simulink model "task_5_model"  (R2021b)
settings: Solver=FixedStepAuto  StartTime=0.0  StopTime=2  FixedStep=0.001  RelTol=1e-3
settings Model: Creator=den  LastModifiedBy=den

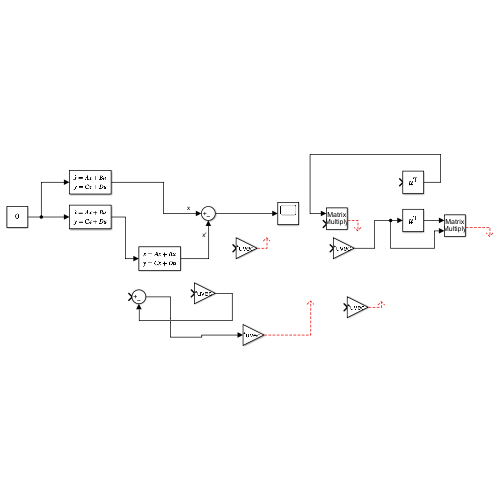
[thumbnail: Simulink's stored preview of the top-level diagram]
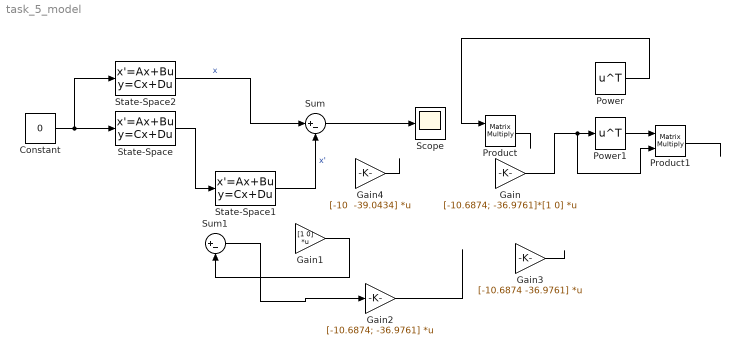
== system task_5_model ==
  Constant : Constant  Value=0
  Gain : Gain  Gain=[-10.6874; -36.9761]*[1 0]  Multiplication=Matrix(K*u) (u vector)
  Gain1 : Gain  Gain=[1 0]  Multiplication=Matrix(K*u) (u vector)
  Gain2 : Gain  Gain=[-10.6874; -36.9761]  Multiplication=Matrix(K*u) (u vector)
  Gain3 : Gain  Gain=[-10.6874 -36.9761]  Multiplication=Matrix(K*u) (u vector)
  Gain4 : Gain  Gain="[-10  -39.0434]"  Multiplication=Matrix(K*u) (u vector)
  Power : Math  Operator=transpose  SaturateOnIntegerOverflow=on
  Power1 : Math  Operator=transpose  SaturateOnIntegerOverflow=on
  Product : Product  Multiplication=Matrix(*)
  Product1 : Product  Multiplication=Matrix(*)
  Scope : Scope
  State-Space : StateSpace  A=[0 1; 0 0]  B=[0; 0]  C=[1 0]  D=0  InitialCondition=[1; 0]
  State-Space1 : StateSpace  A="[-10    1.0000;  -39.0434        0]"  B="[10.0000;   39.0434]"  C=[1 0; 0 1]  D=[0;0]  InitialCondition=[0;-1]
  State-Space2 : StateSpace  A=[0 1; 0 0]  B=[0; 0]  C=[1 0; 0 1]  D=[0;0]  InitialCondition=[1; 0]
  Sum : Sum  Inputs=|+-
  Sum1 : Sum  Inputs=|+-
  wires:
  State-Space/1 -> State-Space1/1
  State-Space1/1 -> Sum/2  "x'"
  Constant/1 -> State-Space2/1, State-Space/1
  State-Space2/1 -> Sum/1  "x"
  Power/1 -> Product/1
  Product/1 -> ?
  Gain/1 -> Product1/2, Power1/1
  Power1/1 -> Product1/1
  Product1/1 -> ?
  Gain1/1 -> Sum1/2
  Sum1/1 -> Gain2/1
  Gain2/1 -> ?
  Gain3/1 -> ?
  Sum/1 -> Scope/1
  Gain4/1 -> ?
